simulink model "inpguitest"  (Simulink 8.3)
settings: Solver=FixedStepDiscrete  StartTime=0.0  StopTime=inf  RelTol=1e-3
settings Model: Creator=nskandan  LastModifiedBy=Aluno  CovSFcnEnable=on
settings OptimizationCC: InitFltsAndDblsToZero=on
settings DebuggingCC: SaveWithParameterizedLinksMsg=none  SignalResolutionControl=TryResolveAllWithWarning  FcnCallInpInsideContextMsg=UseLocalSettings  FrameProcessingCompatibilityMsg=error  StateNameClashWarn=none
settings GRTTargetCC: TargetFcnLib=ansi_tfl_tmw.mat

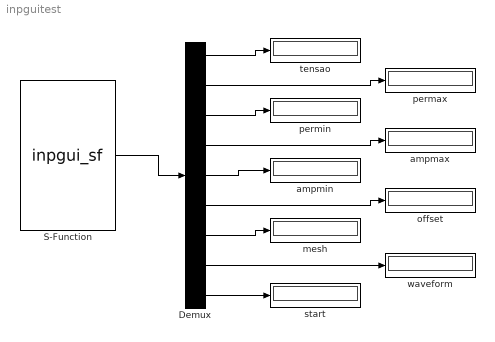
== system inpguitest ==
  Demux : Demux  Outputs=9
  S-Function : S-Function  FunctionName=inpgui_sf  Parameters=0.005  EnableBusSupport=off
  ampmax : Display
  ampmin : Display
  mesh : Display
  offset : Display
  permax : Display
  permin : Display
  start : Display
  tensao : Display
  waveform : Display
  wires:
  S-Function/1 -> Demux/1
  Demux/1 -> tensao/1
  Demux/2 -> permax/1
  Demux/3 -> permin/1
  Demux/4 -> ampmax/1
  Demux/5 -> ampmin/1
  Demux/6 -> offset/1
  Demux/7 -> mesh/1
  Demux/8 -> waveform/1
  Demux/9 -> start/1
